simulink model "obsv_model"  (R2021b)
settings: Solver=FixedStepAuto  StartTime=0.0  StopTime=1  FixedStep=0.01  RelTol=1e-3
values from neighbouring files (symbols this model uses):
  A = [0 1 0 0; -K/M 0 K/M 0; 0 0 0 1; K/M 0 -K/M 0]    [desafio2.m]
  Areal = [0 1 0 0; -K/M 0 K/M 0; 0 0 0 1; K/M 0 -K/M 0]    [desafio2.m]
  B = [0 0; 1/M 0; 0 0; 0 1/M]    [desafio2.m]
  Breal = [0 0; 1/M 0; 0 0; 0 1/M]    [desafio2.m]
  C = [1 0 0 0; 0 0 1 0]    [desafio2.m]
  D = [0 0; 0 0]    [desafio2.m]
  Wo = obsv_gramm(A, C, [0 Tf])    [desafio2.m]    (also in obsv_gramm.m = integral(dWo, time_interval(1), time_interval(2), 'ArrayValu)
  x0 = [2; 0; 1; 0]    [desafio2.m]    (also in obsv_estimate_x0.m = Wo\integral(dx0, 0, Tf, 'ArrayValued', true))
  zero = [0; 0; 0; 0]    [desafio2.m]
settings Model: Creator=Murillo  LastModifiedBy=Murillo

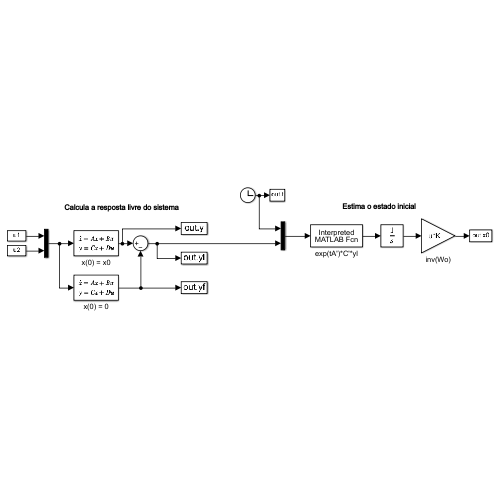
[thumbnail: Simulink's stored preview of the top-level diagram]
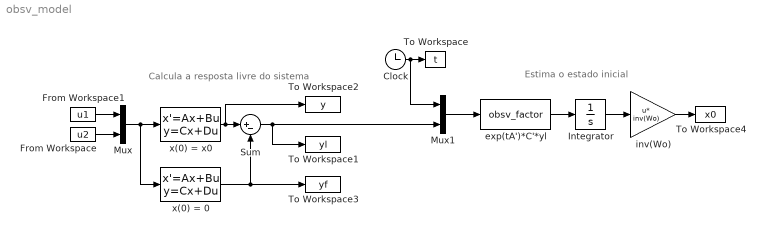
== system obsv_model ==
  note: Estima o estado inicial
  note: Calcula a resposta livre do sistema
  Clock : Clock
  From Workspace : FromWorkspace  VariableName=u2
  From Workspace1 : FromWorkspace  VariableName=u1
  Integrator : Integrator
  Mux : Mux  Inputs=2
  Mux1 : Mux  Inputs=2
  Sum : Sum  Inputs=|+-
  To Workspace : ToWorkspace  VariableName=t  SampleTime=-1
      settings: Save2DSignal=2-D array (concatenate along first dimension)
  To Workspace1 : ToWorkspace  VariableName=yl  SampleTime=-1
      settings: Save2DSignal=2-D array (concatenate along first dimension)
  To Workspace2 : ToWorkspace  VariableName=y  SampleTime=-1
      settings: Save2DSignal=2-D array (concatenate along first dimension)
  To Workspace3 : ToWorkspace  VariableName=yf  SampleTime=-1
      settings: Save2DSignal=2-D array (concatenate along first dimension)
  To Workspace4 : ToWorkspace  VariableName=x0  SampleTime=-1
      settings: Save2DSignal=2-D array (concatenate along first dimension)
  exp(tA')*C'*yl : MATLABFcn  MATLABFcn=obsv_factor
  inv(Wo) : Gain  Gain=inv(Wo)  Multiplication=Matrix(u*K)
  x(0) = 0 : StateSpace  A=A  B=B  C=C  D=D  InitialCondition=zero
  x(0) = x0 : StateSpace  A=Areal  B=Breal  C=C  D=D  InitialCondition=x0
  wires:
  Mux/1 -> x(0) = 0/1, x(0) = x0/1
  From Workspace1/1 -> Mux/1
  From Workspace/1 -> Mux/2
  Clock/1 -> Mux1/1, To Workspace/1
  x(0) = 0/1 -> Sum/2, To Workspace3/1
  x(0) = x0/1 -> To Workspace2/1, Sum/1
  Sum/1 -> To Workspace1/1, Mux1/2
  inv(Wo)/1 -> To Workspace4/1
  Mux1/1 -> exp(tA')*C'*yl/1
  exp(tA')*C'*yl/1 -> Integrator/1
  Integrator/1 -> inv(Wo)/1
